simulink model "robotprueba3"  (R2018a)
settings: Solver=VariableStepAuto  StartTime=0.0  StopTime=200  FixedStep=0.01  RelTol=1e-6
model workspace: external: MATLAB File C:\Users\PC\Desktop\10 SEMESTRE\inteligencia artificial\simscape prueba2\robotprueba3_DataFile.m (data not in the file)
values from neighbouring files (symbols this model uses):
  m = (str2double(get(handles.edit8,'String'))/100)*p    [Reconocerpatron.m]
  N = rand(1)    [seleccion.m]
  s =     [s.mat]
  X = timetable(X,'TimeStep',seconds(0.1))    [Reconocerpatron.m]
  Y = timetable(Y,'TimeStep',seconds(0.1))    [Reconocerpatron.m]    (also in cruzamiento.m = zeros (x1,n); mutacion.m = zeros (x1,n))
undefined symbols (not defined in the file or in its folder): smiData, Z
libraries: sm_lib x72, nesl_utility x35, fl_lib x3
(part 3 of 3)

== matlab function robotprueba3/Control/MATLAB Function ==
  data: x input; velR output; y input; phi input; velL output; pxd input; pyd input; l input
function [velR,velL] = fcn(x,y,phi,pxd,pyd,l)
K1=0.5;
K2=0.5;
q2=0.5;

phid=45*(pi/180);
phi=90*(pi/180)+phi;
iota=sqrt((pxd-x)^2+(pyd-y)^2);
dseta=atan2((pyd-y),(pxd-x))-phi;
psi=atan2((pyd-y),(pxd-x))-phid;

if l==0
uref=double(K1*cos(dseta)*iota);
wref=double(K2*dseta+(K1/dseta)*cos(dseta)*sin(dseta)*(dseta+q2*psi));
else
    uref=0;
    wref=0;
end

velR=double((2*uref+wref*0.29184)/(2*0.032));
velL=double((2*uref-wref*0.29184)/(2*0.032));
